simulink model "left_vs_center_PWM_DAC"  (R2018b)
settings: Solver=VariableStepAuto  StartTime=0.0  StopTime=0.01  RelTol=1e-3
undefined symbols (not defined in the file or in its folder): f_pwm
libraries: simulink x1
settings Model: Creator=Marcel  LastModifiedBy=Marcel

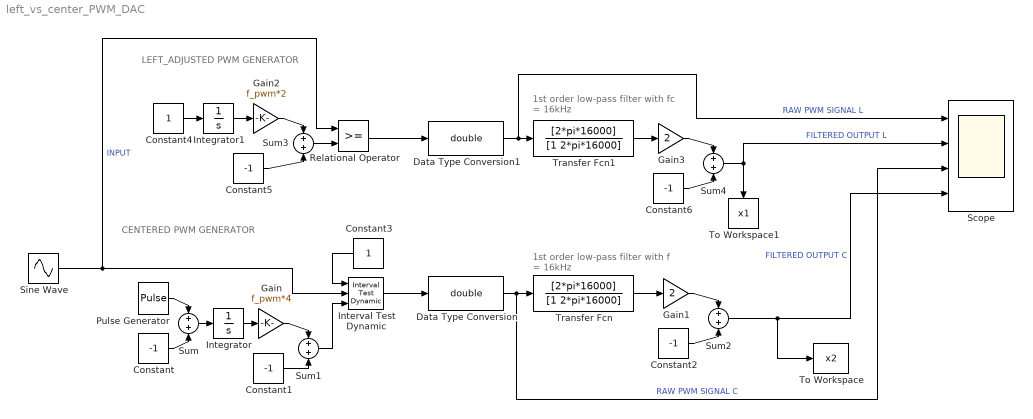
== system left_vs_center_PWM_DAC ==
  note: 1st order low-pass filter
      | with f = 16kHz
  note: CENTERED PWM
      | GENERATOR
  note: 1st order low-pass filter
      | with fc = 16kHz
  note: LEFT_ADJUSTED PWM
      | GENERATOR
  Constant{,1..2,5..6} (5 alike) : Constant  Value=-1
  Constant3 : Constant
  Constant4 : Constant
  Data Type Conversion : DataTypeConversion  OutMin=[0]  OutMax=[1]  OutDataTypeStr=double
  Data Type Conversion1 : DataTypeConversion  OutMin=[0]  OutMax=[1]  OutDataTypeStr=double
  Gain : Gain  Gain=f_pwm*4
  Gain1 : Gain  Gain=2
  Gain2 : Gain  Gain=f_pwm*2
  Gain3 : Gain  Gain=2
  Integrator : Integrator
  Integrator1 : Integrator  WrapState=on  WrappedStateUpperValue=1/(1*f_pwm)  WrappedStateLowerValue=0
  Interval Test Dynamic : simulink/Logic and Bit Operations/Interval Test Dynamic  IntervalClosedRight=on  IntervalClosedLeft=on  OutDataTypeStr=boolean
      settings: SourceProductName=Simulink  SourceProductBaseCode=SL
  Pulse Generator : DiscretePulseGenerator  PulseType=Time based  Amplitude=2  Period=1/f_pwm  PulseWidth=50
  Relational Operator : RelationalOperator  OutDataTypeStr=boolean  RndMeth=Simplest
  Scope : Scope  NumInputPorts=4
  Sine Wave : Sin  Frequency=2*pi*5e3  SampleTime=0
  Sum{,1..4} (5 alike) : Sum  Inputs=2
  To Workspace : ToWorkspace  VariableName=x2  SaveFormat=Structure With Time  SampleTime=1e-7
  To Workspace1 : ToWorkspace  VariableName=x1  SaveFormat=Structure With Time  SampleTime=1e-7
  Transfer Fcn : TransferFcn  Numerator=[2*pi*16000]  Denominator=[1 2*pi*16000]
  Transfer Fcn1 : TransferFcn  Numerator=[2*pi*16000]  Denominator=[1 2*pi*16000]
  wires:
  Constant3/1 -> Interval Test Dynamic/1
  Interval Test Dynamic/1 -> Data Type Conversion/1
  Constant/1 -> Sum/2
  Constant1/1 -> Sum1/2
  Gain1/1 -> Sum2/1
  Sum2/1 -> Scope/4, To Workspace/1  "FILTERED OUTPUT C"
  Integrator/1 -> Gain/1
  Gain/1 -> Sum1/1
  Data Type Conversion/1 -> Scope/3, Transfer Fcn/1  "RAW PWM SIGNAL C"
  Constant2/1 -> Sum2/2
  Sum/1 -> Integrator/1
  Transfer Fcn/1 -> Gain1/1
  Sine Wave/1 -> Relational Operator/1, Interval Test Dynamic/2  "INPUT"
  Pulse Generator/1 -> Sum/1
  Constant4/1 -> Integrator1/1
  Transfer Fcn1/1 -> Gain3/1
  Constant6/1 -> Sum4/2
  Relational Operator/1 -> Data Type Conversion1/1
  Data Type Conversion1/1 -> Scope/1, Transfer Fcn1/1  "RAW PWM SIGNAL L"
  Sum3/1 -> Relational Operator/2
  Gain3/1 -> Sum4/1
  Sum4/1 -> To Workspace1/1, Scope/2  "FILTERED OUTPUT L"
  Integrator1/1 -> Gain2/1
  Gain2/1 -> Sum3/1
  Constant5/1 -> Sum3/2
  Sum1/1 -> Interval Test Dynamic/3
